simulink model "sulfitadornn"  (R2021a)
settings: Solver=ode45  StartTime=0.0  StopTime=2000  MaxStep=10  RelTol=1e-3  AbsTol=1e-3  EnableMultiTasking=on
model workspace (MAT data in the model file):
  socvcb : containers.Map (value not decoded)
values from neighbouring files (symbols this model uses):
  Kd = K(2)    [Funcion_FitnessObjetivo.m]    (also in Planta.m = 16.9826)
  Ke = K(1)    [Funcion_FitnessObjetivo.m]    (also in Planta.m = 18.2675)
  Ku = K(3)    [Funcion_FitnessObjetivo.m]    (also in Planta.m = 8.63912)
libraries: neural x198, fuzblock x1
(part 4 of 6)

== system sulfitadornn/Cascade-Forward Neural Network/Layer 3/Delays 1 ==
  "p{3}" : Inport  PortDimensions=1
      mask Display: e = 0.06;c1 = [120 230 180]/255;c2 = ([120 230 180]+0)/(256+128);c3 = ([120 230 180]+128)/(256+128);patch([0 1 1 0],[0 0 1 1],c1);patch([0 1 1 1-e 1-e 0+e],[0 0 1 1-e 0+e 0+e],c2);patch([0 0 1 1-e 0+e 0+e],[0 1 1 1-e 1-e 0+e],c3);plot([0 1 1 0 0],[0 0 1 1 0]);
  mux : Mux  Inputs=1
      mask Display: e = 0.06;c1 = [120 150 230]/255;c2 = ([120 150 230]+0)/383;c3 = ([120 150 230]+128)/383;patch([0 1 1 0],[0 0 1 1],c1);patch([0 1 1 1-e 1-e 0+e],[0 0 1 1-e 0+e 0+e],c2);patch([0 0 1 1-e 0+e 0+e],[0 1 1 1-e 1-e 0+e],c3);plot([0 1 1 0 0],[0 0 1 1 0]);disp('Mux')
  "pd{3,1}" : Outport
      mask Display: e = 0.06;c1 = [120 230 180]/255;c2 = ([120 230 180]+0)/(256+128);c3 = ([120 230 180]+128)/(256+128);patch([0 1 1 0],[0 0 1 1],c1);patch([0 1 1 1-e 1-e 0+e],[0 0 1 1-e 0+e 0+e],c2);patch([0 0 1 1-e 0+e 0+e],[0 1 1 1-e 1-e 0+e],c3);plot([0 1 1 0 0],[0 0 1 1 0]);
  wires:
  "p{3}"/1 -> mux/1
  mux/1 -> "pd{3,1}"/1

== system sulfitadornn/Cascade-Forward Neural Network/Layer 3/Delays 2 ==
  "p{3}" : Inport  PortDimensions=20
      mask Display: e = 0.06;c1 = [120 230 180]/255;c2 = ([120 230 180]+0)/(256+128);c3 = ([120 230 180]+128)/(256+128);patch([0 1 1 0],[0 0 1 1],c1);patch([0 1 1 1-e 1-e 0+e],[0 0 1 1-e 0+e 0+e],c2);patch([0 0 1 1-e 0+e 0+e],[0 1 1 1-e 1-e 0+e],c3);plot([0 1 1 0 0],[0 0 1 1 0]);
  mux : Mux  Inputs=1
      mask Display: e = 0.06;c1 = [120 150 230]/255;c2 = ([120 150 230]+0)/383;c3 = ([120 150 230]+128)/383;patch([0 1 1 0],[0 0 1 1],c1);patch([0 1 1 1-e 1-e 0+e],[0 0 1 1-e 0+e 0+e],c2);patch([0 0 1 1-e 0+e 0+e],[0 1 1 1-e 1-e 0+e],c3);plot([0 1 1 0 0],[0 0 1 1 0]);disp('Mux')
  "pd{3,1}" : Outport
      mask Display: e = 0.06;c1 = [120 230 180]/255;c2 = ([120 230 180]+0)/(256+128);c3 = ([120 230 180]+128)/(256+128);patch([0 1 1 0],[0 0 1 1],c1);patch([0 1 1 1-e 1-e 0+e],[0 0 1 1-e 0+e 0+e],c2);patch([0 0 1 1-e 0+e 0+e],[0 1 1 1-e 1-e 0+e],c3);plot([0 1 1 0 0],[0 0 1 1 0]);
  wires:
  "p{3}"/1 -> mux/1
  mux/1 -> "pd{3,1}"/1

== system sulfitadornn/Cascade-Forward Neural Network/Layer 3/Delays 3 ==
  "p{3}" : Inport  PortDimensions=50
      mask Display: e = 0.06;c1 = [120 230 180]/255;c2 = ([120 230 180]+0)/(256+128);c3 = ([120 230 180]+128)/(256+128);patch([0 1 1 0],[0 0 1 1],c1);patch([0 1 1 1-e 1-e 0+e],[0 0 1 1-e 0+e 0+e],c2);patch([0 0 1 1-e 0+e 0+e],[0 1 1 1-e 1-e 0+e],c3);plot([0 1 1 0 0],[0 0 1 1 0]);
  mux : Mux  Inputs=1
      mask Display: e = 0.06;c1 = [120 150 230]/255;c2 = ([120 150 230]+0)/383;c3 = ([120 150 230]+128)/383;patch([0 1 1 0],[0 0 1 1],c1);patch([0 1 1 1-e 1-e 0+e],[0 0 1 1-e 0+e 0+e],c2);patch([0 0 1 1-e 0+e 0+e],[0 1 1 1-e 1-e 0+e],c3);plot([0 1 1 0 0],[0 0 1 1 0]);disp('Mux')
  "pd{3,2}" : Outport
      mask Display: e = 0.06;c1 = [120 230 180]/255;c2 = ([120 230 180]+0)/(256+128);c3 = ([120 230 180]+128)/(256+128);patch([0 1 1 0],[0 0 1 1],c1);patch([0 1 1 1-e 1-e 0+e],[0 0 1 1-e 0+e 0+e],c2);patch([0 0 1 1-e 0+e 0+e],[0 1 1 1-e 1-e 0+e],c3);plot([0 1 1 0 0],[0 0 1 1 0]);
  wires:
  "p{3}"/1 -> mux/1
  mux/1 -> "pd{3,2}"/1

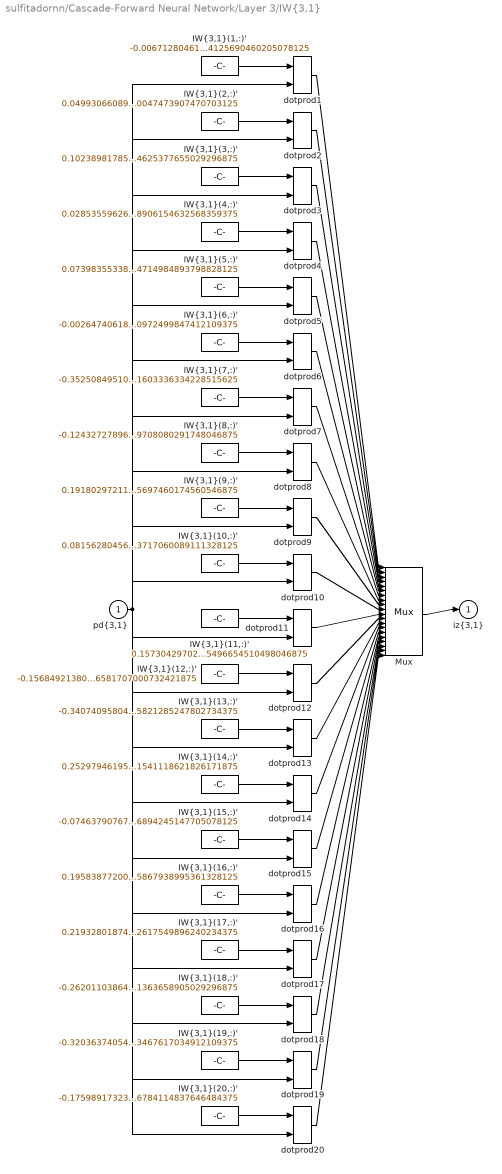
== system sulfitadornn/Cascade-Forward Neural Network/Layer 3/IW{3,1} ==
  "pd{3,1}" : Inport  PortDimensions=1
      mask Display: e = 0.06;c1 = [120 230 180]/255;c2 = ([120 230 180]+0)/(256+128);c3 = ([120 230 180]+128)/(256+128);patch([0 1 1 0],[0 0 1 1],c1);patch([0 1 1 1-e 1-e 0+e],[0 0 1 1-e 0+e 0+e],c2);patch([0 0 1 1-e 0+e 0+e],[0 1 1 1-e 1-e 0+e],c3);plot([0 1 1 0 0],[0 0 1 1 0]);
  "IW{3,1}(1,:)'" : Constant  Value=-0.006712804616653825391658916288406544481404125690460205078125
      mask Display: e = 0.06;c1 = [120 150 230]/255;c2 = ([120 150 230]+0)/383;c3 = ([120 150 230]+128)/383;patch([0 1 1 0],[0 0 1 1],c1);patch([0 1 1 1-e 1-e 0+e],[0 0 1 1-e 0+e 0+e],c2);patch([0 0 1 1-e 0+e 0+e],[0 1 1 1-e 1-e 0+e],c3);plot([0 1 1 0 0],[0 0 1 1 0]);disp('Weights');
  "IW{3,1}(10,:)'" : Constant  Value=0.0815628045672582846492559838225133717060089111328125
      mask Display: e = 0.06;c1 = [120 150 230]/255;c2 = ([120 150 230]+0)/383;c3 = ([120 150 230]+128)/383;patch([0 1 1 0],[0 0 1 1],c1);patch([0 1 1 1-e 1-e 0+e],[0 0 1 1-e 0+e 0+e],c2);patch([0 0 1 1-e 0+e 0+e],[0 1 1 1-e 1-e 0+e],c3);plot([0 1 1 0 0],[0 0 1 1 0]);disp('Weights');
  "IW{3,1}(11,:)'" : Constant  Value=0.157304297026638006951060333449277095496654510498046875
      mask Display: e = 0.06;c1 = [120 150 230]/255;c2 = ([120 150 230]+0)/383;c3 = ([120 150 230]+128)/383;patch([0 1 1 0],[0 0 1 1],c1);patch([0 1 1 1-e 1-e 0+e],[0 0 1 1-e 0+e 0+e],c2);patch([0 0 1 1-e 0+e 0+e],[0 1 1 1-e 1-e 0+e],c3);plot([0 1 1 0 0],[0 0 1 1 0]);disp('Weights');
  "IW{3,1}(12,:)'" : Constant  Value=-0.1568492138048602491107175183060462586581707000732421875
      mask Display: e = 0.06;c1 = [120 150 230]/255;c2 = ([120 150 230]+0)/383;c3 = ([120 150 230]+128)/383;patch([0 1 1 0],[0 0 1 1],c1);patch([0 1 1 1-e 1-e 0+e],[0 0 1 1-e 0+e 0+e],c2);patch([0 0 1 1-e 0+e 0+e],[0 1 1 1-e 1-e 0+e],c3);plot([0 1 1 0 0],[0 0 1 1 0]);disp('Weights');
  "IW{3,1}(13,:)'" : Constant  Value=-0.340740958045182562585750929429195821285247802734375
      mask Display: e = 0.06;c1 = [120 150 230]/255;c2 = ([120 150 230]+0)/383;c3 = ([120 150 230]+128)/383;patch([0 1 1 0],[0 0 1 1],c1);patch([0 1 1 1-e 1-e 0+e],[0 0 1 1-e 0+e 0+e],c2);patch([0 0 1 1-e 0+e 0+e],[0 1 1 1-e 1-e 0+e],c3);plot([0 1 1 0 0],[0 0 1 1 0]);disp('Weights');
  "IW{3,1}(14,:)'" : Constant  Value=0.252979461955771867121001150735537521541118621826171875
      mask Display: e = 0.06;c1 = [120 150 230]/255;c2 = ([120 150 230]+0)/383;c3 = ([120 150 230]+128)/383;patch([0 1 1 0],[0 0 1 1],c1);patch([0 1 1 1-e 1-e 0+e],[0 0 1 1-e 0+e 0+e],c2);patch([0 0 1 1-e 0+e 0+e],[0 1 1 1-e 1-e 0+e],c3);plot([0 1 1 0 0],[0 0 1 1 0]);disp('Weights');
  "IW{3,1}(15,:)'" : Constant  Value=-0.0746379076798149576621455025815521366894245147705078125
      mask Display: e = 0.06;c1 = [120 150 230]/255;c2 = ([120 150 230]+0)/383;c3 = ([120 150 230]+128)/383;patch([0 1 1 0],[0 0 1 1],c1);patch([0 1 1 1-e 1-e 0+e],[0 0 1 1-e 0+e 0+e],c2);patch([0 0 1 1-e 0+e 0+e],[0 1 1 1-e 1-e 0+e],c3);plot([0 1 1 0 0],[0 0 1 1 0]);disp('Weights');
  "IW{3,1}(16,:)'" : Constant  Value=0.1958387720043663904334607650525867938995361328125
      mask Display: e = 0.06;c1 = [120 150 230]/255;c2 = ([120 150 230]+0)/383;c3 = ([120 150 230]+128)/383;patch([0 1 1 0],[0 0 1 1],c1);patch([0 1 1 1-e 1-e 0+e],[0 0 1 1-e 0+e 0+e],c2);patch([0 0 1 1-e 0+e 0+e],[0 1 1 1-e 1-e 0+e],c3);plot([0 1 1 0 0],[0 0 1 1 0]);disp('Weights');
  "IW{3,1}(17,:)'" : Constant  Value=0.2193280187462836872125393483656807802617549896240234375
      mask Display: e = 0.06;c1 = [120 150 230]/255;c2 = ([120 150 230]+0)/383;c3 = ([120 150 230]+128)/383;patch([0 1 1 0],[0 0 1 1],c1);patch([0 1 1 1-e 1-e 0+e],[0 0 1 1-e 0+e 0+e],c2);patch([0 0 1 1-e 0+e 0+e],[0 1 1 1-e 1-e 0+e],c3);plot([0 1 1 0 0],[0 0 1 1 0]);disp('Weights');
  "IW{3,1}(18,:)'" : Constant  Value=-0.262011038643771232425905282070743851363658905029296875
      mask Display: e = 0.06;c1 = [120 150 230]/255;c2 = ([120 150 230]+0)/383;c3 = ([120 150 230]+128)/383;patch([0 1 1 0],[0 0 1 1],c1);patch([0 1 1 1-e 1-e 0+e],[0 0 1 1-e 0+e 0+e],c2);patch([0 0 1 1-e 0+e 0+e],[0 1 1 1-e 1-e 0+e],c3);plot([0 1 1 0 0],[0 0 1 1 0]);disp('Weights');
  "IW{3,1}(19,:)'" : Constant  Value=-0.320363740546288189303680837838328443467617034912109375
      mask Display: e = 0.06;c1 = [120 150 230]/255;c2 = ([120 150 230]+0)/383;c3 = ([120 150 230]+128)/383;patch([0 1 1 0],[0 0 1 1],c1);patch([0 1 1 1-e 1-e 0+e],[0 0 1 1-e 0+e 0+e],c2);patch([0 0 1 1-e 0+e 0+e],[0 1 1 1-e 1-e 0+e],c3);plot([0 1 1 0 0],[0 0 1 1 0]);disp('Weights');
  "IW{3,1}(2,:)'" : Constant  Value=0.049930660899312695466534250954282470047473907470703125
      mask Display: e = 0.06;c1 = [120 150 230]/255;c2 = ([120 150 230]+0)/383;c3 = ([120 150 230]+128)/383;patch([0 1 1 0],[0 0 1 1],c1);patch([0 1 1 1-e 1-e 0+e],[0 0 1 1-e 0+e 0+e],c2);patch([0 0 1 1-e 0+e 0+e],[0 1 1 1-e 1-e 0+e],c3);plot([0 1 1 0 0],[0 0 1 1 0]);disp('Weights');
  "IW{3,1}(20,:)'" : Constant  Value=-0.1759891732384103180120149545473395846784114837646484375
      mask Display: e = 0.06;c1 = [120 150 230]/255;c2 = ([120 150 230]+0)/383;c3 = ([120 150 230]+128)/383;patch([0 1 1 0],[0 0 1 1],c1);patch([0 1 1 1-e 1-e 0+e],[0 0 1 1-e 0+e 0+e],c2);patch([0 0 1 1-e 0+e 0+e],[0 1 1 1-e 1-e 0+e],c3);plot([0 1 1 0 0],[0 0 1 1 0]);disp('Weights');
  "IW{3,1}(3,:)'" : Constant  Value=0.1023898178523887370072742442062008194625377655029296875
      mask Display: e = 0.06;c1 = [120 150 230]/255;c2 = ([120 150 230]+0)/383;c3 = ([120 150 230]+128)/383;patch([0 1 1 0],[0 0 1 1],c1);patch([0 1 1 1-e 1-e 0+e],[0 0 1 1-e 0+e 0+e],c2);patch([0 0 1 1-e 0+e 0+e],[0 1 1 1-e 1-e 0+e],c3);plot([0 1 1 0 0],[0 0 1 1 0]);disp('Weights');
  "IW{3,1}(4,:)'" : Constant  Value=0.02853559626558753448133387564666918478906154632568359375
      mask Display: e = 0.06;c1 = [120 150 230]/255;c2 = ([120 150 230]+0)/383;c3 = ([120 150 230]+128)/383;patch([0 1 1 0],[0 0 1 1],c1);patch([0 1 1 1-e 1-e 0+e],[0 0 1 1-e 0+e 0+e],c2);patch([0 0 1 1-e 0+e 0+e],[0 1 1 1-e 1-e 0+e],c3);plot([0 1 1 0 0],[0 0 1 1 0]);disp('Weights');
  "IW{3,1}(5,:)'" : Constant  Value=0.07398355338020130844700616989939589984714984893798828125
      mask Display: e = 0.06;c1 = [120 150 230]/255;c2 = ([120 150 230]+0)/383;c3 = ([120 150 230]+128)/383;patch([0 1 1 0],[0 0 1 1],c1);patch([0 1 1 1-e 1-e 0+e],[0 0 1 1-e 0+e 0+e],c2);patch([0 0 1 1-e 0+e 0+e],[0 1 1 1-e 1-e 0+e],c3);plot([0 1 1 0 0],[0 0 1 1 0]);disp('Weights');
  "IW{3,1}(6,:)'" : Constant  Value=-0.0026474061885173052165176610373009680188260972499847412109375
      mask Display: e = 0.06;c1 = [120 150 230]/255;c2 = ([120 150 230]+0)/383;c3 = ([120 150 230]+128)/383;patch([0 1 1 0],[0 0 1 1],c1);patch([0 1 1 1-e 1-e 0+e],[0 0 1 1-e 0+e 0+e],c2);patch([0 0 1 1-e 0+e 0+e],[0 1 1 1-e 1-e 0+e],c3);plot([0 1 1 0 0],[0 0 1 1 0]);disp('Weights');
  "IW{3,1}(7,:)'" : Constant  Value=-0.352508495102680952104634570787311531603336334228515625
      mask Display: e = 0.06;c1 = [120 150 230]/255;c2 = ([120 150 230]+0)/383;c3 = ([120 150 230]+128)/383;patch([0 1 1 0],[0 0 1 1],c1);patch([0 1 1 1-e 1-e 0+e],[0 0 1 1-e 0+e 0+e],c2);patch([0 0 1 1-e 0+e 0+e],[0 1 1 1-e 1-e 0+e],c3);plot([0 1 1 0 0],[0 0 1 1 0]);disp('Weights');
  "IW{3,1}(8,:)'" : Constant  Value=-0.124327278964688925366743887934717349708080291748046875
      mask Display: e = 0.06;c1 = [120 150 230]/255;c2 = ([120 150 230]+0)/383;c3 = ([120 150 230]+128)/383;patch([0 1 1 0],[0 0 1 1],c1);patch([0 1 1 1-e 1-e 0+e],[0 0 1 1-e 0+e 0+e],c2);patch([0 0 1 1-e 0+e 0+e],[0 1 1 1-e 1-e 0+e],c3);plot([0 1 1 0 0],[0 0 1 1 0]);disp('Weights');
  "IW{3,1}(9,:)'" : Constant  Value=0.191802972117595782464150033774785697460174560546875
      mask Display: e = 0.06;c1 = [120 150 230]/255;c2 = ([120 150 230]+0)/383;c3 = ([120 150 230]+128)/383;patch([0 1 1 0],[0 0 1 1],c1);patch([0 1 1 1-e 1-e 0+e],[0 0 1 1-e 0+e 0+e],c2);patch([0 0 1 1-e 0+e 0+e],[0 1 1 1-e 1-e 0+e],c3);plot([0 1 1 0 0],[0 0 1 1 0]);disp('Weights');
  Mux : Mux  Inputs=20
      mask Display: e = 0.06;c1 = [120 150 230]/255;c2 = ([120 150 230]+0)/383;c3 = ([120 150 230]+128)/383;patch([0 1 1 0],[0 0 1 1],c1);patch([0 1 1 1-e 1-e 0+e],[0 0 1 1-e 0+e 0+e],c2);patch([0 0 1 1-e 0+e 0+e],[0 1 1 1-e 1-e 0+e],c3);plot([0 1 1 0 0],[0 0 1 1 0]);disp('Mux');
  dotprod{1..20} (20 alike) : neural/Weight Functions/dotprod
  "iz{3,1}" : Outport
      mask Display: e = 0.06;c1 = [120 230 180]/255;c2 = ([120 230 180]+0)/(256+128);c3 = ([120 230 180]+128)/(256+128);patch([0 1 1 0],[0 0 1 1],c1);patch([0 1 1 1-e 1-e 0+e],[0 0 1 1-e 0+e 0+e],c2);patch([0 0 1 1-e 0+e 0+e],[0 1 1 1-e 1-e 0+e],c3);plot([0 1 1 0 0],[0 0 1 1 0]);
  wires:
  "IW{3,1}(1,:)'"/1 -> dotprod1/1
  "pd{3,1}"/1 -> dotprod1/2, dotprod2/2, dotprod3/2, dotprod4/2, dotprod5/2, dotprod6/2, dotprod7/2, dotprod8/2, dotprod9/2, dotprod10/2, dotprod11/2, dotprod12/2, dotprod13/2, dotprod14/2, dotprod15/2, dotprod16/2, dotprod17/2, dotprod18/2, dotprod19/2, dotprod20/2
  dotprod1/1 -> Mux/1
  "IW{3,1}(2,:)'"/1 -> dotprod2/1
  dotprod2/1 -> Mux/2
  "IW{3,1}(3,:)'"/1 -> dotprod3/1
  dotprod3/1 -> Mux/3
  "IW{3,1}(4,:)'"/1 -> dotprod4/1
  dotprod4/1 -> Mux/4
  "IW{3,1}(5,:)'"/1 -> dotprod5/1
  dotprod5/1 -> Mux/5
  "IW{3,1}(6,:)'"/1 -> dotprod6/1
  dotprod6/1 -> Mux/6
  "IW{3,1}(7,:)'"/1 -> dotprod7/1
  dotprod7/1 -> Mux/7
  "IW{3,1}(8,:)'"/1 -> dotprod8/1
  dotprod8/1 -> Mux/8
  "IW{3,1}(9,:)'"/1 -> dotprod9/1
  dotprod9/1 -> Mux/9
  "IW{3,1}(10,:)'"/1 -> dotprod10/1
  dotprod10/1 -> Mux/10
  "IW{3,1}(11,:)'"/1 -> dotprod11/1
  dotprod11/1 -> Mux/11
  "IW{3,1}(12,:)'"/1 -> dotprod12/1
  dotprod12/1 -> Mux/12
  "IW{3,1}(13,:)'"/1 -> dotprod13/1
  dotprod13/1 -> Mux/13
  "IW{3,1}(14,:)'"/1 -> dotprod14/1
  dotprod14/1 -> Mux/14
  "IW{3,1}(15,:)'"/1 -> dotprod15/1
  dotprod15/1 -> Mux/15
  "IW{3,1}(16,:)'"/1 -> dotprod16/1
  dotprod16/1 -> Mux/16
  "IW{3,1}(17,:)'"/1 -> dotprod17/1
  dotprod17/1 -> Mux/17
  "IW{3,1}(18,:)'"/1 -> dotprod18/1
  dotprod18/1 -> Mux/18
  "IW{3,1}(19,:)'"/1 -> dotprod19/1
  dotprod19/1 -> Mux/19
  "IW{3,1}(20,:)'"/1 -> dotprod20/1
  dotprod20/1 -> Mux/20
  Mux/1 -> "iz{3,1}"/1

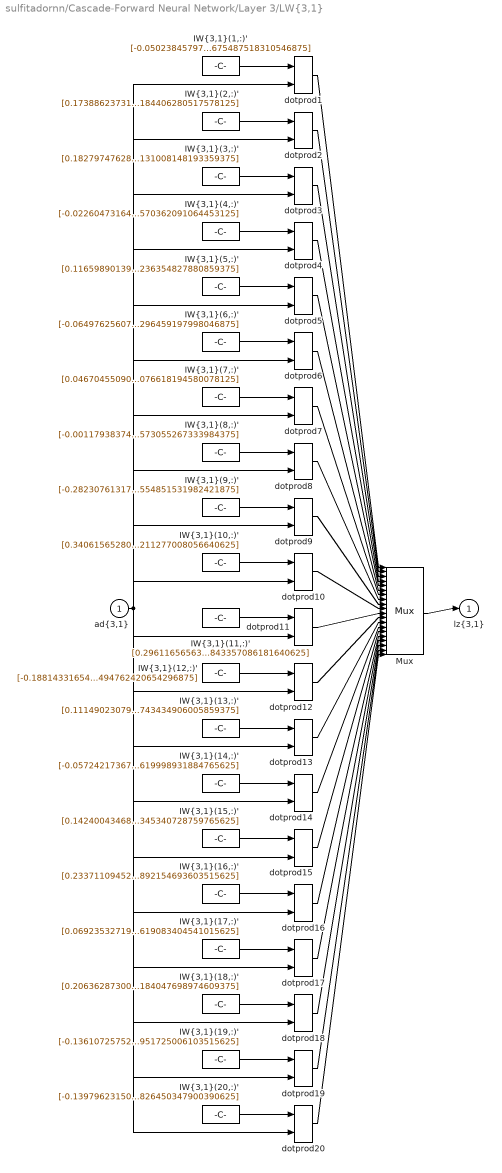
== system sulfitadornn/Cascade-Forward Neural Network/Layer 3/LW{3,1} ==
  "ad{3,1}" : Inport  PortDimensions=20
      mask Display: e = 0.06;c1 = [120 230 180]/255;c2 = ([120 230 180]+0)/(256+128);c3 = ([120 230 180]+128)/(256+128);patch([0 1 1 0],[0 0 1 1],c1);patch([0 1 1 1-e 1-e 0+e],[0 0 1 1-e 0+e 0+e],c2);patch([0 0 1 1-e 0+e 0+e],[0 1 1 1-e 1-e 0+e],c3);plot([0 1 1 0 0],[0 0 1 1 0]);
  "IW{3,1}(1,:)'" : Constant  Value=[-0.050238457971350798658694003506752778775990009307861328125;-0.1987608553391727872483585315421805717051029205322265625;0.06486119259859453312078159115117159672081470489501953125;-0.09956195857627771206299627237967797555029392242431640625;0.166675237462831582480049519290332682430744171142578125;0.210430671637947985797012506736791692674160003662109375;-0.1016075309434289752896773961765575222671031951904296875;0.2011272310160348852914324879748164676129817962646484375;0.011094198924655691851359762267748010344803333282470703125;0.2156872604483713040668391158760641701519489288330078125;0.236318452354081831590093543127295561134815216064453125;-0.2279872083819105832436235914428834803402423858642578125;-0.05831137494195061388158052295693778432905673980712890625;-0.240427671210178051097727802698500454425811767578125;-0.09942218082048219496282825957678142003715038299560546875;-0.2223127366856580688914135635059210471808910369873046875;-0.25362067823928458043525324683287180960178375244140625;-0.214627781284847773957125127708422951400279998779296875;0.00801043031624557554104537615558001562021672725677490234375;0.08528205883395212349995517797651700675487518310546875]
      mask Display: e = 0.06;c1 = [120 150 230]/255;c2 = ([120 150 230]+0)/383;c3 = ([120 150 230]+128)/383;patch([0 1 1 0],[0 0 1 1],c1);patch([0 1 1 1-e 1-e 0+e],[0 0 1 1-e 0+e 0+e],c2);patch([0 0 1 1-e 0+e 0+e],[0 1 1 1-e 1-e 0+e],c3);plot([0 1 1 0 0],[0 0 1 1 0]);disp('weights');
  "IW{3,1}(10,:)'" : Constant  Value=[0.340615652807070568020009204701636917889118194580078125;0.271193794147551126005879496005945838987827301025390625;-0.04734028119052535732436126636457629501819610595703125;-0.023415825722512641215988793419455760158598423004150390625;0.044020614650967272718506961837192648090422153472900390625;-0.047701684489258988630666635799570940434932708740234375;0.06705448010901694788632454446997144259512424468994140625;0.193181047690101304059595577200525440275669097900390625;0.0545839196803517279210637980213505215942859649658203125;0.2483425586462379153207535864567034877836704254150390625;-0.0459172709836890569068401646291022188961505889892578125;-0.247482490869180338233235261213849298655986785888671875;-0.34628726123949482573749492075876332819461822509765625;0.2130527676341088805234136316357762552797794342041015625;0.2658099211055093835653906353400088846683502197265625;0.001927587359713524295390385532300570048391819000244140625;0.1483776320946338100892347711123875342309474945068359375;-0.1772512620065896660204174395403242669999599456787109375;-0.23142854541088997422093598288483917713165283203125;0.0778184877364266613941623518257983960211277008056640625]
      mask Display: e = 0.06;c1 = [120 150 230]/255;c2 = ([120 150 230]+0)/383;c3 = ([120 150 230]+128)/383;patch([0 1 1 0],[0 0 1 1],c1);patch([0 1 1 1-e 1-e 0+e],[0 0 1 1-e 0+e 0+e],c2);patch([0 0 1 1-e 0+e 0+e],[0 1 1 1-e 1-e 0+e],c3);plot([0 1 1 0 0],[0 0 1 1 0]);disp('weights');
  "IW{3,1}(11,:)'" : Constant  Value=[0.296116565632517148021207731289905495941638946533203125;-0.12430044889208595459972883645605179481208324432373046875;-0.32269019378460950253639794027549214661121368408203125;-0.150867342919740521356430917876423336565494537353515625;0.1241396770833722296156764741681399755179882049560546875;-0.05818343377068403710072885814952314831316471099853515625;-0.09371583122978512092604574945653439499437808990478515625;-0.07501822408558765642450083532821736298501491546630859375;0.17115357239135875477842319014598615467548370361328125;-0.21720816858859015585636598189012147486209869384765625;0.00708733479934551234558082200010176165960729122161865234375;0.095713663814094462889414671735721640288829803466796875;0.13561692068241859576716024093911983072757720947265625;0.31284880606764053911916789729730226099491119384765625;0.3463857081808676685596992683713324368000030517578125;0.24722323105056898118192520996672101318836212158203125;0.051129430166967936022270890816798782907426357269287109375;-0.00025931501159031180615832656854991000727750360965728759765625;0.04707797996580199983984726941343978978693485260009765625;-0.031428367761382448863916039272226043976843357086181640625]
      mask Display: e = 0.06;c1 = [120 150 230]/255;c2 = ([120 150 230]+0)/383;c3 = ([120 150 230]+128)/383;patch([0 1 1 0],[0 0 1 1],c1);patch([0 1 1 1-e 1-e 0+e],[0 0 1 1-e 0+e 0+e],c2);patch([0 0 1 1-e 0+e 0+e],[0 1 1 1-e 1-e 0+e],c3);plot([0 1 1 0 0],[0 0 1 1 0]);disp('weights');
  "IW{3,1}(12,:)'" : Constant  Value=[-0.188143316548090189233022329062805511057376861572265625;0.339005537492877817573599941169959492981433868408203125;0.2089092024277520442954170221128151752054691314697265625;-0.497114673710640830872620199443190358579158782958984375;-0.1671627785438183078081664234559866599738597869873046875;-0.028330504841724148124004756255089887417852878570556640625;-0.149629995804633375566794484257115982472896575927734375;-0.046068188518664399122570785038988105952739715576171875;0.227542032076130718021289567332132719457149505615234375;0.28404117311510013177411337892408482730388641357421875;0.164228704867812214107658519424148835241794586181640625;-0.282702645142464181748920282188919372856616973876953125;-0.055985735520321593117198943900802987627685070037841796875;-0.0891382184455582760040925904831965453922748565673828125;-0.143594675915075964400813290922087617218494415283203125;-0.0114601986215487061659956680159666575491428375244140625;0.129492395641607582756904548659804277122020721435546875;-0.023214868623468602748527445100990007631480693817138671875;0.07987681389774252405100440910246106795966625213623046875;-0.279291857846286351030329342393088154494762420654296875]
      mask Display: e = 0.06;c1 = [120 150 230]/255;c2 = ([120 150 230]+0)/383;c3 = ([120 150 230]+128)/383;patch([0 1 1 0],[0 0 1 1],c1);patch([0 1 1 1-e 1-e 0+e],[0 0 1 1-e 0+e 0+e],c2);patch([0 0 1 1-e 0+e 0+e],[0 1 1 1-e 1-e 0+e],c3);plot([0 1 1 0 0],[0 0 1 1 0]);disp('weights');
  "IW{3,1}(13,:)'" : Constant  Value=[0.111490230793025890676517519750632345676422119140625;0.30913398951312609508335071950568817555904388427734375;0.0304223401836052793900666557647127774544060230255126953125;0.0179086786640663721270616548508769483305513858795166015625;0.2376244296241381004364257023553363978862762451171875;0.1540952350261357850502719202268053777515888214111328125;0.01418803941584514775875458525433714385144412517547607421875;-0.0303362893037333429535618023464849102310836315155029296875;0.1259718952039507733342560413802857510745525360107421875;-0.1671265595120978719734239348326809704303741455078125;0.1465929617606653023731411167318583466112613677978515625;0.017697350249739181304864388266651076264679431915283203125;-0.1588534702958212807555327117370325140655040740966796875;0.215601425566729953953171161629143171012401580810546875;-0.0144129585208821638098175554887347971089184284210205078125;-0.24700532528955176925222758654854260385036468505859375;-0.1139413197667918653532836970043717883527278900146484375;-0.11624976339066382668985255577354109846055507659912109375;-0.075953803199640568255546213549678213894367218017578125;0.267129281058923806480009943697950802743434906005859375]
      mask Display: e = 0.06;c1 = [120 150 230]/255;c2 = ([120 150 230]+0)/383;c3 = ([120 150 230]+128)/383;patch([0 1 1 0],[0 0 1 1],c1);patch([0 1 1 1-e 1-e 0+e],[0 0 1 1-e 0+e 0+e],c2);patch([0 0 1 1-e 0+e 0+e],[0 1 1 1-e 1-e 0+e],c3);plot([0 1 1 0 0],[0 0 1 1 0]);disp('weights');
  "IW{3,1}(14,:)'" : Constant  Value=[-0.05724217367614554963228812312081572599709033966064453125;-0.0017692817531776024696232862964961896068416535854339599609375;0.1722816265983490857660598294387455098330974578857421875;-0.330579922524667890737504194476059637963771820068359375;0.1431149934814071877919872122220112942159175872802734375;-0.11669706988449819740072399554264848120510578155517578125;-0.048805073331960470428558807043373235501348972320556640625;-0.1664160722291646854475999361966387368738651275634765625;0.05429785982675559841137413741307682357728481292724609375;-0.0612984540506069930376753518430632539093494415283203125;0.19368369419242059681351975086727179586887359619140625;0.250043398272049299801977895185700617730617523193359375;-0.2200450949879960427235658926292671822011470794677734375;-0.3489730987140973184068570844829082489013671875;0.1615695917481372034796294201441924087703227996826171875;0.278526510686644412917445379207492806017398834228515625;-0.09549238540416855880454960470160585828125476837158203125;-0.16530926330783313193961703291279263794422149658203125;0.113228270754819615451225445212912745773792266845703125;0.112299356330821942240305588711635209619998931884765625]
      mask Display: e = 0.06;c1 = [120 150 230]/255;c2 = ([120 150 230]+0)/383;c3 = ([120 150 230]+128)/383;patch([0 1 1 0],[0 0 1 1],c1);patch([0 1 1 1-e 1-e 0+e],[0 0 1 1-e 0+e 0+e],c2);patch([0 0 1 1-e 0+e 0+e],[0 1 1 1-e 1-e 0+e],c3);plot([0 1 1 0 0],[0 0 1 1 0]);disp('weights');
  "IW{3,1}(15,:)'" : Constant  Value=[0.142400434686191790234488507849164307117462158203125;-0.000927280228178838290299668134508692673989571630954742431640625;0.231994672566345039310675701926811598241329193115234375;0.0742487997872301741519862616769387386739253997802734375;0.252965091872070946266148894210346043109893798828125;0.1179545023005535708815472162314108572900295257568359375;0.1585367574357315623156949868644005618989467620849609375;0.2068149581670273295941342439618892967700958251953125;0.1776033843860521932445095671937451697885990142822265625;-0.21351586786096776737764457720913924276828765869140625;-0.285467001178421220242142908318783156573772430419921875;-0.1920307939588484502646537066539167426526546478271484375;0.25043121230052090009365883815917186439037322998046875;0.041442304905415616733677097727195359766483306884765625;0.115160872806775393950573516121949069201946258544921875;0.052925422366147507891032120141971972770988941192626953125;-0.0462179006434662309477090502696228213608264923095703125;0.219650506810115386802095827079028822481632232666015625;0.230084950377532904131072655218304134905338287353515625;0.07256135262330455637513892952483729459345340728759765625]
      mask Display: e = 0.06;c1 = [120 150 230]/255;c2 = ([120 150 230]+0)/383;c3 = ([120 150 230]+128)/383;patch([0 1 1 0],[0 0 1 1],c1);patch([0 1 1 1-e 1-e 0+e],[0 0 1 1-e 0+e 0+e],c2);patch([0 0 1 1-e 0+e 0+e],[0 1 1 1-e 1-e 0+e],c3);plot([0 1 1 0 0],[0 0 1 1 0]);disp('weights');
  "IW{3,1}(16,:)'" : Constant  Value=[0.2337110945234564252093178993163746781647205352783203125;0.1880009127193456863746945373350172303617000579833984375;-0.280691520740291189373039060228620655834674835205078125;0.0638900589578248467859111769939772784709930419921875;-0.266170720179681741246469073303160257637500762939453125;-0.25118643151199548935181837805430404841899871826171875;0.0430868638446823271070940108984359540045261383056640625;-0.146971096549477986403786644586944021284580230712890625;-0.0256523609045540661177664532033304567448794841766357421875;-0.0671019181913639906067459151017828844487667083740234375;-0.0858265521691053134833992999119800515472888946533203125;-0.233016751118262976927297813745099119842052459716796875;-0.2414406308363861441979025812543113715946674346923828125;0.11861444312402870393530207593357772566378116607666015625;0.05051682258193394836620626620060647837817668914794921875;-0.15937339489399404701686080443323589861392974853515625;0.1621785138510260793065498319265316240489482879638671875;-0.261036196383064356130176975057111121714115142822265625;-0.1815991431862007121633695305717992596328258514404296875;0.0828804682997338615368931868943036533892154693603515625]
      mask Display: e = 0.06;c1 = [120 150 230]/255;c2 = ([120 150 230]+0)/383;c3 = ([120 150 230]+128)/383;patch([0 1 1 0],[0 0 1 1],c1);patch([0 1 1 1-e 1-e 0+e],[0 0 1 1-e 0+e 0+e],c2);patch([0 0 1 1-e 0+e 0+e],[0 1 1 1-e 1-e 0+e],c3);plot([0 1 1 0 0],[0 0 1 1 0]);disp('weights');
  "IW{3,1}(17,:)'" : Constant  Value=[0.06923532719743728802708204739246866665780544281005859375;0.2210626308224466207708047704727505333721637725830078125;-0.2118983521597826158444632937971618957817554473876953125;-0.042717781469628963997298143340231035836040973663330078125;-0.18286188485948418058768538685399107635021209716796875;0.02464660308306400315903061937206075526773929595947265625;0.335079249273968871047912898575305007398128509521484375;0.22555855579382189102233269295538775622844696044921875;-0.258807126747546079048589717785944230854511260986328125;-0.1452964622936454841539699600616586394608020782470703125;-0.11571856066246648253592610444684396497905254364013671875;0.06477999613454266114587198899243958294391632080078125;-0.050403288223355102726230825282982550561428070068359375;0.108399848529982356648559971290524117648601531982421875;-0.1925872161966506179719971214581164531409740447998046875;0.349085412941065487135716693956055678427219390869140625;-0.40399355327108998903185010931338183581829071044921875;0.001810740320646785084246488395365304313600063323974609375;0.268316408543034234934765436264569871127605438232421875;0.034451985301630884406254295981852919794619083404541015625]
      mask Display: e = 0.06;c1 = [120 150 230]/255;c2 = ([120 150 230]+0)/383;c3 = ([120 150 230]+128)/383;patch([0 1 1 0],[0 0 1 1],c1);patch([0 1 1 1-e 1-e 0+e],[0 0 1 1-e 0+e 0+e],c2);patch([0 0 1 1-e 0+e 0+e],[0 1 1 1-e 1-e 0+e],c3);plot([0 1 1 0 0],[0 0 1 1 0]);disp('weights');
  "IW{3,1}(18,:)'" : Constant  Value=[0.2063628730069952676995370666190865449607372283935546875;0.1597495957976387825905106865320703946053981781005859375;-0.1775194237529131024988515719087445177137851715087890625;0.262896194862685117499268017127178609371185302734375;0.1244662751708714154563750753368367440998554229736328125;-0.11400493779028088303650889656637446023523807525634765625;0.0934309082526383338773712239344604313373565673828125;-0.284163398200881378574678137738374061882495880126953125;0.07837899007053832078906197011747281067073345184326171875;-0.296840483890893402918464971662615425884723663330078125;-0.1184737058746887783389212245310773141682147979736328125;0.2457670060097275344102030203430331312119960784912109375;-0.05520379015432129443663455958812846802175045013427734375;-0.0116858639060495213268797698447087896056473255157470703125;0.249833082117048521642033165335305966436862945556640625;0.057541071792609123358719358520829700864851474761962890625;-0.04967807321249685659214634370073326863348484039306640625;0.01533799915455853930812413210560407605953514575958251953125;0.24703311450745413235807745877536945044994354248046875;-0.19143921978708566822291459175175987184047698974609375]
      mask Display: e = 0.06;c1 = [120 150 230]/255;c2 = ([120 150 230]+0)/383;c3 = ([120 150 230]+128)/383;patch([0 1 1 0],[0 0 1 1],c1);patch([0 1 1 1-e 1-e 0+e],[0 0 1 1-e 0+e 0+e],c2);patch([0 0 1 1-e 0+e 0+e],[0 1 1 1-e 1-e 0+e],c3);plot([0 1 1 0 0],[0 0 1 1 0]);disp('weights');
  "IW{3,1}(19,:)'" : Constant  Value=[-0.1361072575259265615699177942587994039058685302734375;0.03705682928311397617004985249877790920436382293701171875;-0.29285077714539908821933522631297819316387176513671875;-5.5649654842142813604422002526916912756860256195068359375e-06;-0.2271051088041904642000901048959349282085895538330078125;-0.1401583720462077631285779943937086500227451324462890625;0.1826818784285774988074280145156080834567546844482421875;-0.0290811421297938917096548294694002834148705005645751953125;0.16239648680755525145258388874935917556285858154296875;0.04172567436963368903146687216576538048684597015380859375;-0.1990331476437632030052071741010877303779125213623046875;0.2311626327226120325430969160152017138898372650146484375;0.493540727704047277324406195475603453814983367919921875;-0.07311679344385234313730137500897399149835109710693359375;0.09090859744219027815947953286013216711580753326416015625;0.00651811092529592205069288723962017684243619441986083984375;0.312199037775425125573747209273278713226318359375;0.30960178967129003968494771470432169735431671142578125;0.12243741509292029034927651309772045351564884185791015625;-0.085481214958216311661232111873687244951725006103515625]
      mask Display: e = 0.06;c1 = [120 150 230]/255;c2 = ([120 150 230]+0)/383;c3 = ([120 150 230]+128)/383;patch([0 1 1 0],[0 0 1 1],c1);patch([0 1 1 1-e 1-e 0+e],[0 0 1 1-e 0+e 0+e],c2);patch([0 0 1 1-e 0+e 0+e],[0 1 1 1-e 1-e 0+e],c3);plot([0 1 1 0 0],[0 0 1 1 0]);disp('weights');
  "IW{3,1}(2,:)'" : Constant  Value=[0.1738862373159533181166125359595753252506256103515625;0.2446215135441689725315228542967815883457660675048828125;-0.2532684054617242441764801696990616619586944580078125;-0.030115160915681150888278949651066795922815799713134765625;0.020788897863507786734071913770094397477805614471435546875;-0.21292391420780754085484431925578974187374114990234375;-0.09752859079438254419347487100822036154568195343017578125;0.07709130667586534813029430779351969249546527862548828125;-0.03335154890665281701700450867065228521823883056640625;0.1018451650007712039336382758847321383655071258544921875;-0.1783287453318992132889064805567613802850246429443359375;-0.19055788747656909887240317402756772935390472412109375;0.19790970668902552187518040227587334811687469482421875;0.23946754396396141562064485697192139923572540283203125;0.2473944430774386582516655153085594065487384796142578125;0.02513405501991326784771985103361657820641994476318359375;-0.277332983695371793064765597591758705675601959228515625;-0.31698053890911281893494333417038433253765106201171875;0.0715835918852185393301823523870552890002727508544921875;0.13196838549179468191852038216893561184406280517578125]
      mask Display: e = 0.06;c1 = [120 150 230]/255;c2 = ([120 150 230]+0)/383;c3 = ([120 150 230]+128)/383;patch([0 1 1 0],[0 0 1 1],c1);patch([0 1 1 1-e 1-e 0+e],[0 0 1 1-e 0+e 0+e],c2);patch([0 0 1 1-e 0+e 0+e],[0 1 1 1-e 1-e 0+e],c3);plot([0 1 1 0 0],[0 0 1 1 0]);disp('weights');
  "IW{3,1}(20,:)'" : Constant  Value=[-0.1397962315030993052378249785760999657213687896728515625;0.1795590254343092662114855784238898195326328277587890625;0.2349955390003729271963806013445719145238399505615234375;-0.2382318930994415662194541027929517440497875213623046875;0.1318443749371664142078230952392914332449436187744140625;0.189951066005663637970002355359611101448535919189453125;0.171063045433668181605213476359494961798191070556640625;0.237734528956585255965450187431997619569301605224609375;0.0860157286286169220357322728887083940207958221435546875;0.1731919719702606774713871118365204893052577972412109375;0.04732703707561604355991136117154383100569248199462890625;-0.10878668486826929828747978490355308167636394500732421875;-0.306550587751032665995154502525110729038715362548828125;-0.042389664728047338204675043016322888433933258056640625;0.08051448735330356265560425299554481171071529388427734375;-0.1357784406596825588220411873408011160790920257568359375;-0.4018684636559022305135613351012580096721649169921875;-0.053586608032069139861963691373603069223463535308837890625;-0.21757331904107946041193599739926867187023162841796875;-0.18551244588224680143184741609729826450347900390625]
      mask Display: e = 0.06;c1 = [120 150 230]/255;c2 = ([120 150 230]+0)/383;c3 = ([120 150 230]+128)/383;patch([0 1 1 0],[0 0 1 1],c1);patch([0 1 1 1-e 1-e 0+e],[0 0 1 1-e 0+e 0+e],c2);patch([0 0 1 1-e 0+e 0+e],[0 1 1 1-e 1-e 0+e],c3);plot([0 1 1 0 0],[0 0 1 1 0]);disp('weights');
  "IW{3,1}(3,:)'" : Constant  Value=[0.1827974762855704427000347322973539121448993682861328125;-0.06649657698829113117167111113303690217435359954833984375;-0.162188602141460247452187104499898850917816162109375;-0.291363483300896231042997897020541131496429443359375;-0.1344288718383888359131361767140333540737628936767578125;0.181845948190571593539033301567542366683483123779296875;0.1402486428468214807452341119642369449138641357421875;-0.252617566520019209974634577520191669464111328125;-0.2741050869084367125338985715643502771854400634765625;-0.06732952722096230413484363452880643308162689208984375;-0.2310859784662222804474396298246574588119983673095703125;-0.039314405369878617502177320375267299823462963104248046875;-0.0904042991858686750816787025541998445987701416015625;-0.0770757988074767530495279288516030646860599517822265625;0.07755737445819503583788190326231415383517742156982421875;0.198123385931463502629412687383592128753662109375;-0.154954005476050316048031163518317043781280517578125;-0.1672955992857134421836207138767349533736705780029296875;-0.16043787801156217387443803090718574821949005126953125;0.01449760858777442672218338515222058049403131008148193359375]
      mask Display: e = 0.06;c1 = [120 150 230]/255;c2 = ([120 150 230]+0)/383;c3 = ([120 150 230]+128)/383;patch([0 1 1 0],[0 0 1 1],c1);patch([0 1 1 1-e 1-e 0+e],[0 0 1 1-e 0+e 0+e],c2);patch([0 0 1 1-e 0+e 0+e],[0 1 1 1-e 1-e 0+e],c3);plot([0 1 1 0 0],[0 0 1 1 0]);disp('weights');
  "IW{3,1}(4,:)'" : Constant  Value=[-0.022604731649914035218618124645217903889715671539306640625;-0.0183031738099542484743409431757754646241664886474609375;0.25523781756466001890970574095263145864009857177734375;-0.25510335862893562808295655486290343105792999267578125;0.04367957255919781289765779774825205095112323760986328125;0.2173170025730443433165106625892804004251956939697265625;-0.2621621890088718931366429387708194553852081298828125;-0.050427183194529601184541434122365899384021759033203125;-0.009599718342626649414395245685227564536035060882568359375;0.02389409159414636329987757790149771608412265777587890625;-0.20620652631331937154612887752591632306575775146484375;0.0223248938224050279266474916539664263837039470672607421875;0.2037365346653391140474553822059533558785915374755859375;-0.1846227168949541030951166931117768399417400360107421875;0.274987790165666101671604337752796709537506103515625;-0.1035527872975099683561239771734108217060565948486328125;-0.153559698688788326403908968131872825324535369873046875;-0.263952340560187070916953189225750975310802459716796875;0.23921198537061771904888018980273045599460601806640625;-0.0791218449765265507966915947690722532570362091064453125]
      mask Display: e = 0.06;c1 = [120 150 230]/255;c2 = ([120 150 230]+0)/383;c3 = ([120 150 230]+128)/383;patch([0 1 1 0],[0 0 1 1],c1);patch([0 1 1 1-e 1-e 0+e],[0 0 1 1-e 0+e 0+e],c2);patch([0 0 1 1-e 0+e 0+e],[0 1 1 1-e 1-e 0+e],c3);plot([0 1 1 0 0],[0 0 1 1 0]);disp('weights');
  "IW{3,1}(5,:)'" : Constant  Value=[0.11659890139298910438636625030994764529168605804443359375;0.1968134984865404224496643337261048145592212677001953125;0.072014792892126477941161510898382402956485748291015625;0.209274606076973623824954984229407273232936859130859375;0.0290448961784668148455867964230492361821234226226806640625;0.2975635663994002921839410191751085221767425537109375;-0.034511152301140650411337418290713685564696788787841796875;-0.262991346970014971962115168935270048677921295166015625;0.04260885246400870907113045404912554658949375152587890625;-0.180322132597017681376883047050796449184417724609375;-0.2317432986939381434066120846182457171380519866943359375;0.128666516064014302411777634915779344737529754638671875;0.1777720342318790669455808028942556120455265045166015625;0.12361594540582714063514657709674793295562267303466796875;0.20173346588276130919581419220776297152042388916015625;0.24649709000197106423257764618028886616230010986328125;0.09099277200022275191582110664967331103980541229248046875;0.254680667064608068361764026121818460524082183837890625;0.08667075407563762379226091070449911057949066162109375;-0.271193105915521426307890351381502114236354827880859375]
      mask Display: e = 0.06;c1 = [120 150 230]/255;c2 = ([120 150 230]+0)/383;c3 = ([120 150 230]+128)/383;patch([0 1 1 0],[0 0 1 1],c1);patch([0 1 1 1-e 1-e 0+e],[0 0 1 1-e 0+e 0+e],c2);patch([0 0 1 1-e 0+e 0+e],[0 1 1 1-e 1-e 0+e],c3);plot([0 1 1 0 0],[0 0 1 1 0]);disp('weights');
  "IW{3,1}(6,:)'" : Constant  Value=[-0.06497625607859076890537863846475374884903430938720703125;0.0508390099389399996443472673490759916603565216064453125;0.187899930737764175869841665189596824347972869873046875;-0.1269942647665458224093271155652473680675029754638671875;0.1125094207551522729193749228215892799198627471923828125;0.291410488806726875044006419557263143360614776611328125;-0.266055264668957625051604054533527232706546783447265625;0.232648689413668507963706133523373864591121673583984375;-0.2200132846630475091931344877593801356852054595947265625;-0.0387737924162266101024698627952602691948413848876953125;-0.133816418243036305835147459220024757087230682373046875;-0.1864136001771884154631919727762578986585140228271484375;0.1506176347238125934335783995265956036746501922607421875;-0.277629495866465736408912334809429012238979339599609375;0.2537800044077818117926881313906051218509674072265625;-0.060991375619490868775773861898414907045662403106689453125;0.14797245555716564968662396495346911251544952392578125;0.28160950328435052636422142313676886260509490966796875;0.269162222715155829977362600402557291090488433837890625;-0.12089885331906284615666180570769938640296459197998046875]
      mask Display: e = 0.06;c1 = [120 150 230]/255;c2 = ([120 150 230]+0)/383;c3 = ([120 150 230]+128)/383;patch([0 1 1 0],[0 0 1 1],c1);patch([0 1 1 1-e 1-e 0+e],[0 0 1 1-e 0+e 0+e],c2);patch([0 0 1 1-e 0+e 0+e],[0 1 1 1-e 1-e 0+e],c3);plot([0 1 1 0 0],[0 0 1 1 0]);disp('weights');
  "IW{3,1}(7,:)'" : Constant  Value=[0.046704550907768711820455820316055906005203723907470703125;-0.06284471283966863719427919932059012353420257568359375;-0.26324987227244800447323314074310474097728729248046875;0.143956253610660278585697824382805265486240386962890625;0.18987579852175617833864862404880113899707794189453125;0.03381630343020895768102462852766620926558971405029296875;-0.136448161283463875736998716092784889042377471923828125;-0.0885077371629765519145394137012772262096405029296875;-0.037152731449570396138337713409782736562192440032958984375;-0.2336663893179648232578671240844414569437503814697265625;-0.243631140522984790397487131485831923782825469970703125;-0.342612877688796835240481186701799742877483367919921875;0.20492294833005086918120696282130666077136993408203125;0.1948846629287672993502411600275081582367420196533203125;0.2496261739978387905747325703487149439752101898193359375;-0.2354259724576226175951632058058748953044414520263671875;0.2466341280160018190059645348810590803623199462890625;-0.085963058605496966979586659363121725618839263916015625;-0.30274640895093651860037198275676928460597991943359375;-0.0340705361394509076422565385655616410076618194580078125]
      mask Display: e = 0.06;c1 = [120 150 230]/255;c2 = ([120 150 230]+0)/383;c3 = ([120 150 230]+128)/383;patch([0 1 1 0],[0 0 1 1],c1);patch([0 1 1 1-e 1-e 0+e],[0 0 1 1-e 0+e 0+e],c2);patch([0 0 1 1-e 0+e 0+e],[0 1 1 1-e 1-e 0+e],c3);plot([0 1 1 0 0],[0 0 1 1 0]);disp('weights');
  "IW{3,1}(8,:)'" : Constant  Value=[-0.00117938374019573195827792488898921874351799488067626953125;-0.0105137803886011411969025886037343298085033893585205078125;0.05354435060357125297780811479242402128875255584716796875;0.0403348806802489023848323768106638453900814056396484375;-0.2209886122085648330060081434567109681665897369384765625;0.0308207128233830111863067457989018294028937816619873046875;-0.1176858577648235149037958535700454376637935638427734375;-0.256850800397598832969237037104903720319271087646484375;-0.1257213309433363457312538002952351234853267669677734375;0.016818852790801759600203268973928061313927173614501953125;0.054350593178488025569716768359285197220742702484130859375;0.1577747086862592296174767625416279770433902740478515625;-0.03153171190775745647005834371157106943428516387939453125;0.28642235450576902788810684796771965920925140380859375;0.164027841091488324476443949606618843972682952880859375;0.1539875702729178730265857666381634771823883056640625;-0.252275209331435712467595067209913395345211029052734375;0.36513263272456619734640526075963862240314483642578125;0.0610223189306693669653469669356127269566059112548828125;0.2367314021995896577976736807613633573055267333984375]
      mask Display: e = 0.06;c1 = [120 150 230]/255;c2 = ([120 150 230]+0)/383;c3 = ([120 150 230]+128)/383;patch([0 1 1 0],[0 0 1 1],c1);patch([0 1 1 1-e 1-e 0+e],[0 0 1 1-e 0+e 0+e],c2);patch([0 0 1 1-e 0+e 0+e],[0 1 1 1-e 1-e 0+e],c3);plot([0 1 1 0 0],[0 0 1 1 0]);disp('weights');
  "IW{3,1}(9,:)'" : Constant  Value=[-0.28230761317508934471476322869420982897281646728515625;0.1835649031005679165939881158919888548552989959716796875;0.2850977933778502393380449575488455593585968017578125;-0.3108275508770430572980103534064255654811859130859375;-0.035894951542667273558517848641713499091565608978271484375;-0.408428859863175564015591589850373566150665283203125;-0.060096019403743150544272566548897884786128997802734375;-0.185247258866032493695996663518599234521389007568359375;-0.1829805110198828022038952667571720667183399200439453125;-0.08177020004443368017543747328090830706059932708740234375;0.174794316059194654311426120329997502267360687255859375;-0.300285787909106371973422255905461497604846954345703125;0.1374545587846467409320894148549996316432952880859375;0.113975977258436333983127042301930487155914306640625;0.035786730571416604240742032061461941339075565338134765625;0.198917800606052852518956797212013043463230133056640625;-0.038174432200733958431282388801264460198581218719482421875;-0.0894431628083356133895875927919405512511730194091796875;-0.041452689808858800279978140679304488003253936767578125;-0.3580470719728274797688527542049996554851531982421875]
      mask Display: e = 0.06;c1 = [120 150 230]/255;c2 = ([120 150 230]+0)/383;c3 = ([120 150 230]+128)/383;patch([0 1 1 0],[0 0 1 1],c1);patch([0 1 1 1-e 1-e 0+e],[0 0 1 1-e 0+e 0+e],c2);patch([0 0 1 1-e 0+e 0+e],[0 1 1 1-e 1-e 0+e],c3);plot([0 1 1 0 0],[0 0 1 1 0]);disp('weights');
  Mux : Mux  Inputs=20
      mask Display: e = 0.06;c1 = [120 150 230]/255;c2 = ([120 150 230]+0)/383;c3 = ([120 150 230]+128)/383;patch([0 1 1 0],[0 0 1 1],c1);patch([0 1 1 1-e 1-e 0+e],[0 0 1 1-e 0+e 0+e],c2);patch([0 0 1 1-e 0+e 0+e],[0 1 1 1-e 1-e 0+e],c3);plot([0 1 1 0 0],[0 0 1 1 0]);disp('Mux');
  dotprod{1..20} (20 alike) : neural/Weight Functions/dotprod
  "lz{3,1}" : Outport
      mask Display: e = 0.06;c1 = [120 230 180]/255;c2 = ([120 230 180]+0)/(256+128);c3 = ([120 230 180]+128)/(256+128);patch([0 1 1 0],[0 0 1 1],c1);patch([0 1 1 1-e 1-e 0+e],[0 0 1 1-e 0+e 0+e],c2);patch([0 0 1 1-e 0+e 0+e],[0 1 1 1-e 1-e 0+e],c3);plot([0 1 1 0 0],[0 0 1 1 0]);
  wires:
  "IW{3,1}(1,:)'"/1 -> dotprod1/1
  "ad{3,1}"/1 -> dotprod1/2, dotprod2/2, dotprod3/2, dotprod4/2, dotprod5/2, dotprod6/2, dotprod7/2, dotprod8/2, dotprod9/2, dotprod10/2, dotprod11/2, dotprod12/2, dotprod13/2, dotprod14/2, dotprod15/2, dotprod16/2, dotprod17/2, dotprod18/2, dotprod19/2, dotprod20/2
  dotprod1/1 -> Mux/1
  "IW{3,1}(2,:)'"/1 -> dotprod2/1
  dotprod2/1 -> Mux/2
  "IW{3,1}(3,:)'"/1 -> dotprod3/1
  dotprod3/1 -> Mux/3
  "IW{3,1}(4,:)'"/1 -> dotprod4/1
  dotprod4/1 -> Mux/4
  "IW{3,1}(5,:)'"/1 -> dotprod5/1
  dotprod5/1 -> Mux/5
  "IW{3,1}(6,:)'"/1 -> dotprod6/1
  dotprod6/1 -> Mux/6
  "IW{3,1}(7,:)'"/1 -> dotprod7/1
  dotprod7/1 -> Mux/7
  "IW{3,1}(8,:)'"/1 -> dotprod8/1
  dotprod8/1 -> Mux/8
  "IW{3,1}(9,:)'"/1 -> dotprod9/1
  dotprod9/1 -> Mux/9
  "IW{3,1}(10,:)'"/1 -> dotprod10/1
  dotprod10/1 -> Mux/10
  "IW{3,1}(11,:)'"/1 -> dotprod11/1
  dotprod11/1 -> Mux/11
  "IW{3,1}(12,:)'"/1 -> dotprod12/1
  dotprod12/1 -> Mux/12
  "IW{3,1}(13,:)'"/1 -> dotprod13/1
  dotprod13/1 -> Mux/13
  "IW{3,1}(14,:)'"/1 -> dotprod14/1
  dotprod14/1 -> Mux/14
  "IW{3,1}(15,:)'"/1 -> dotprod15/1
  dotprod15/1 -> Mux/15
  "IW{3,1}(16,:)'"/1 -> dotprod16/1
  dotprod16/1 -> Mux/16
  "IW{3,1}(17,:)'"/1 -> dotprod17/1
  dotprod17/1 -> Mux/17
  "IW{3,1}(18,:)'"/1 -> dotprod18/1
  dotprod18/1 -> Mux/18
  "IW{3,1}(19,:)'"/1 -> dotprod19/1
  dotprod19/1 -> Mux/19
  "IW{3,1}(20,:)'"/1 -> dotprod20/1
  dotprod20/1 -> Mux/20
  Mux/1 -> "lz{3,1}"/1
